simulink subsystem "LateralMetrics"  (R2022b)
settings: Solver=VariableStepAuto  StartTime=0.0  StopTime=10.0  RelTol=1e-3
settings Model: Creator=The MathWorks, Inc.  LastModifiedBy=The MathWorks, Inc.
settings SolverCC: MaxZcPerStep=1
settings DebuggingCC: UnconnectedInputMsg=warning  UnconnectedOutputMsg=warning  UnconnectedLineMsg=warning
settings ModelReferenceCC: EnableRefExpFcnMdlSchedulingChecks=on
settings RTWCC: DLArmComputeVersion=19.05

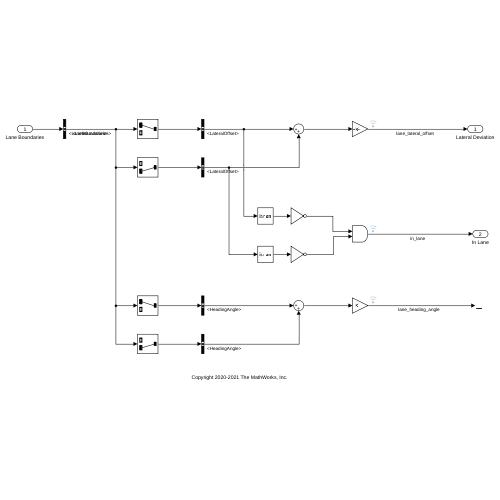
[thumbnail: Simulink's stored preview of the top-level diagram]
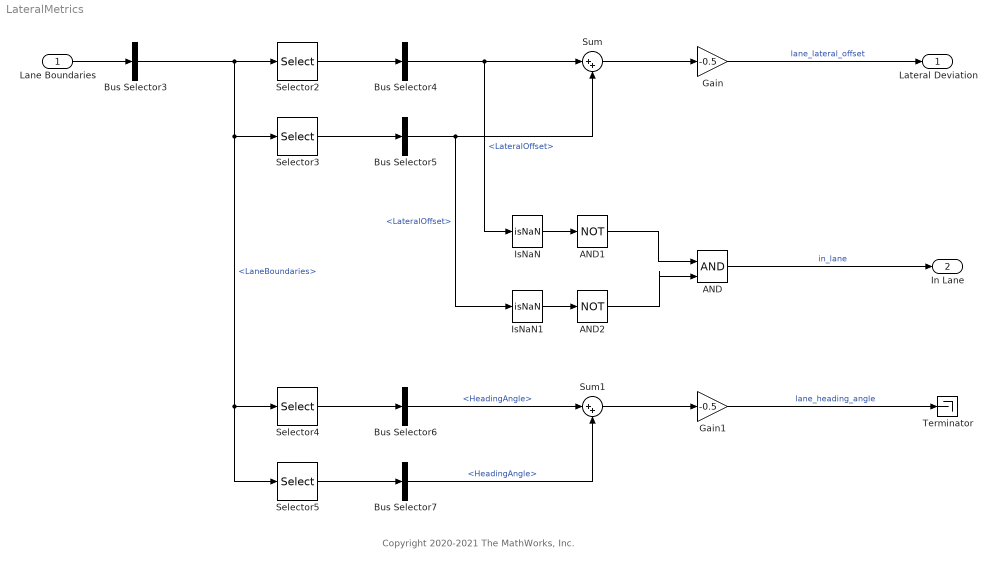
== system LateralMetrics ==
  note: Copyright 2020-2021 The MathWorks, Inc.
  Lane Boundaries : Inport
  AND : Logic  IconShape=distinctive  AllPortsSameDT=off  OutDataTypeStr=boolean
  AND1 : Logic  Operator=NOT  IconShape=distinctive  AllPortsSameDT=off  OutDataTypeStr=boolean
  AND2 : Logic  Operator=NOT  IconShape=distinctive  AllPortsSameDT=off  OutDataTypeStr=boolean
  Bus Selector3 : BusSelector  OutputSignals=LaneBoundaries
  Bus Selector4 : BusSelector  OutputSignals=LateralOffset
  Bus Selector5 : BusSelector  OutputSignals=LateralOffset
  Bus Selector6 : BusSelector  OutputSignals=HeadingAngle
  Bus Selector7 : BusSelector  OutputSignals=HeadingAngle
  Gain : Gain  Gain=-0.5
  Gain1 : Gain  Gain=-0.5
  IsNaN : RelationalOperator  Operator=isNaN  OutDataTypeStr=boolean  RndMeth=Simplest  InputSameDT=off
  IsNaN1 : RelationalOperator  Operator=isNaN  OutDataTypeStr=boolean  RndMeth=Simplest  InputSameDT=off
  Selector2 : Selector  InputPortWidth=2  IndexOptions=Index vector (dialog)  Indices=1  OutputSizes=1
  Selector3 : Selector  InputPortWidth=2  IndexOptions=Index vector (dialog)  Indices=2  OutputSizes=1
  Selector4 : Selector  InputPortWidth=2  IndexOptions=Index vector (dialog)  Indices=1  OutputSizes=1
  Selector5 : Selector  InputPortWidth=2  IndexOptions=Index vector (dialog)  Indices=2  OutputSizes=1
  Sum : Sum  Inputs=|++
  Sum1 : Sum  Inputs=|++
  Terminator : Terminator
  Lateral Deviation : Outport  VectorParamsAs1DForOutWhenUnconnected=off
  In Lane : Outport  Port=2
  wires:
  AND/1 -> In Lane/1  "in_lane"
  IsNaN1/1 -> AND2/1
  IsNaN/1 -> AND1/1
  Sum/1 -> Gain/1
  Bus Selector5/1 -> Sum/2, IsNaN1/1  "<LateralOffset>"
  Selector2/1 -> Bus Selector4/1
  Bus Selector4/1 -> Sum/1, IsNaN/1  "<LateralOffset>"
  Selector3/1 -> Bus Selector5/1
  Lane Boundaries/1 -> Bus Selector3/1
  Gain/1 -> Lateral Deviation/1  "lane_lateral_offset"
  AND1/1 -> AND/1
  AND2/1 -> AND/2
  Selector5/1 -> Bus Selector7/1
  Bus Selector6/1 -> Sum1/1  "<HeadingAngle>"
  Selector4/1 -> Bus Selector6/1
  Bus Selector3/1 -> Selector5/1, Selector4/1, Selector3/1, Selector2/1  "<LaneBoundaries>"
  Sum1/1 -> Gain1/1
  Bus Selector7/1 -> Sum1/2  "<HeadingAngle>"
  Gain1/1 -> Terminator/1  "lane_heading_angle"
